simulink model "ExperimentalCarrier"  (R2015b)
settings: Solver=ode45  StartTime=0.0  StopTime=60  FixedStep=0.001  RelTol=1e-4
model workspace (MAT data in the model file):
  CX = [-0.0973267994662 -0.079334770792 -0.063312708602 -0.0492783817904 -0.0372483838751 -0.0272381795582 -0.0192622767468 -0.0133348794834 -0.00947247058383 -0.00770460619817 -0.00779177365154 -0.010332184952 ... (651 elements, 31x21)]
  CX_P = [0.00223913348595 0.00226279846593 0.00215584206323 0.00191826427785 0.0015500651098 0.00105124455907 0.000421802625665 -0.000338260690416 -0.00122894538917 -0.00225025147061 -0.00340217893471 -0.0046847277815 ... (651 elements, 31x21)]
  CX_Q = [0.566750126524 0.513799273419 0.46074149597 0.407560115115 0.354235092058 0.300738098816 0.247021798665 0.193002362465 0.138579422321 0.0841448328254 0.0156800910173 -0.028587220216 ... (651 elements, 31x21)]
  CX_R = [0.00872473439328 0.00961108484928 0.0104908055113 0.0113660862689 0.0122394567236 0.0131139410899 0.0139934759578 0.0148843304351 0.0158005787982 0.0167844985256 0.0173214701743 0.0192824833308 ... (651 elements, 31x21)]
  CX_d_elevator = [0.029681120923 0.0264274948833 0.0231424780296 0.019826833889 0.0164811360769 0.0131055318554 0.00969907215747 0.00625794011772 0.00277062099267 -0.000820697586383 -0.00752061307428 -0.00815142995882 ... (651 elements, 31x21)]
  CX_d_rudder = [-0.00683814731464 -0.00579287968011 -0.00473313798197 -0.00365917618136 -0.00257115069818 -0.00146908461552 -0.000352779652782 0.000778396676178 0.0019254949791 0.00307845824922 0.00430777388103 0.00587395376473 ... (651 elements, 31x21)]
  CY = [0.0748502535538 0.0755645920384 0.0762601803819 0.076936530444 0.0775935707011 0.0782321665355 0.078855460083 0.0794722913019 0.0801051244106 0.0807983900173 0.0815089407636 0.0810999911453 ... (651 elements, 31x21)]
  CY_P = [0.314314541533 0.314908852342 0.315908686179 0.317314043043 0.319124922936 0.321341325856 0.323963251804 0.32699070078 0.330423672784 0.334262167815 0.338506185874 0.343155726961 ... (651 elements, 31x21)]
  CY_Q = [0.206845108985 0.212153285689 0.217549246201 0.223041221006 0.22863865097 0.234352353828 0.240194164072 0.246174375163 0.252295596359 0.258590970539 0.26593702078 0.276814416222 ... (651 elements, 31x21)]
  CY_R = [-0.299983586918 -0.303050767939 -0.30608450573 -0.309088417238 -0.312066630946 -0.315024477354 -0.317970440697 -0.320921537604 -0.323916102322 -0.327010675103 -0.329661903523 -0.331314720608 ... (651 elements, 31x21)]
  CY_d_elevator = [0.0241602483601 0.024862141616 0.0255735782381 0.0262950172254 0.0270270636195 0.0277705820366 0.0285269750226 0.0292988478742 0.0300914026037 0.030913435532 0.0317596917419 0.0324941126108 ... (651 elements, 31x21)]
  CY_d_rudder = [-0.129392052709 -0.131156233114 -0.132888496587 -0.13458992916 -0.13626179938 -0.137905650351 -0.139523580046 -0.141119005177 -0.142698155317 -0.144262742569 -0.145575423934 -0.146927528452 ... (651 elements, 31x21)]
  CZ = [-0.635288026255 -0.561513437672 -0.486937541039 -0.411613157493 -0.335593450001 -0.258932000134 -0.181683022099 -0.10390236702 -0.025657439009 0.0528154193638 0.128636653723 0.209168379022 ... (651 elements, 31x21)]
  CZ_P = [-0.0426180741921 -0.040371283283 -0.0379977363135 -0.0354974332835 -0.0328703741931 -0.0301165590423 -0.027235987831 -0.0242286605594 -0.0210945772272 -0.0178337378347 -0.0144461423817 -0.0109317908683 ... (651 elements, 31x21)]
  CZ_Q = [6.96025865077 6.98114129849 7.00206820292 7.02304903766 7.04409127039 7.06519952703 7.08637371713 7.10760603499 7.12891815552 7.15129935899 7.15392062661 7.18837906802 ... (651 elements, 31x21)]
  CZ_R = [-0.105405414656 -0.106545289739 -0.107737293614 -0.108987554898 -0.110302712806 -0.111690005069 -0.113157533015 -0.114714527104 -0.116362189514 -0.11786971515 -0.114666901886 -0.118318379275 ... (651 elements, 31x21)]
  CZ_d_elevator = [0.51008994796 0.512918903365 0.515635142398 0.518238988463 0.520730557555 0.523109824579 0.525376856974 0.527532585768 0.529582683355 0.53158310039 0.53222009415 0.532991323176 ... (651 elements, 31x21)]
  CZ_d_rudder = [-0.0994246348718 -0.101114338005 -0.102795749856 -0.104468657243 -0.106132886268 -0.107788391525 -0.109435540346 -0.111075916846 -0.112714334729 -0.114363388416 -0.115472857798 -0.116943666826 ... (651 elements, 31x21)]
  Cl = [-0.0385814765962 -0.0383389644596 -0.0380848835968 -0.0378195009591 -0.0375431159662 -0.0372560730473 -0.0369588021987 -0.0366519368415 -0.0363364206354 -0.0360097812088 -0.0355885143095 -0.0352015390645 ... (651 elements, 31x21)]
  Cl_P = [-0.410096776624 -0.411715869817 -0.413321511523 -0.414913701743 -0.416492440476 -0.418057727723 -0.419609563483 -0.421147947757 -0.422672880544 -0.424184361845 -0.425682391659 -0.427166969987 ... (651 elements, 31x21)]
  Cl_Q = [0.0121734873015 0.0115511634771 0.0109219874117 0.0102856172191 0.00964162351347 0.00898936687588 0.00832771640535 0.00765433243871 0.00696211625156 0.00619409954578 0.00511750960358 0.00438446572798 ... (651 elements, 31x21)]
  Cl_R = [0.0639194118456 0.0641980766094 0.0644722880685 0.0647423901469 0.0650087480028 0.0652717875848 0.0655321272397 0.0657909713502 0.0660509927516 0.066314134037 0.0664428977346 0.0665956593355 ... (651 elements, 31x21)]
  Cl_d_elevator = [-0.00083845092376 -0.000897333841468 -0.000957239499541 -0.00101816580014 -0.00108011314323 -0.00114310126406 -0.00120721661945 -0.00127274325287 -0.00134057483614 -0.00141463059496 -0.00150116458646 -0.00150417720092 ... (651 elements, 31x21)]
  Cl_d_rudder = [0.0120074370195 0.0121224981409 0.0122343776715 0.0123431699853 0.0124489831282 0.0125519544191 0.0126522973225 0.0127504304685 0.0128472820476 0.012944583953 0.0130167454048 0.0130728202844 ... (651 elements, 31x21)]
  Cm = [0.0973465601848 0.0882383997807 0.0791321401801 0.0700083578182 0.060846163509 0.0516235998805 0.0423185376691 0.03291173616 0.0234098703618 0.0141912971055 0.0115389891247 -0.00108731819606 ... (651 elements, 31x21)]
  Cm_P = [0.204940910369 0.202805913545 0.20033190145 0.197518874086 0.194366831451 0.190875773546 0.187045700371 0.182876611925 0.17836850821 0.173521389224 0.168335254967 0.162810105441 ... (651 elements, 31x21)]
  Cm_Q = [-8.8302811579 -8.84673802608 -8.86380445529 -8.8815160128 -8.89990381522 -8.91899396376 -8.93880586357 -8.95935222087 -8.98073821097 -9.00528706826 -8.98625605481 -9.03648930164 ... (651 elements, 31x21)]
  Cm_R = [0.231203964913 0.23319997533 0.235299090374 0.237514849258 0.239861907942 0.242356170567 0.245015146547 0.247857975971 0.250885037596 0.253592063858 0.24580144055 0.252971901877 ... (651 elements, 31x21)]
  Cm_d_elevator = [-1.16934045694 -1.17556162403 -1.1814926709 -1.18713462751 -1.19248809506 -1.19755345312 -1.20233156667 -1.2068260282 -1.21105317786 -1.21514844284 -1.21623242778 -1.21673947768 ... (651 elements, 31x21)]
  Cm_d_rudder = [0.221327907125 0.224938352672 0.228521302045 0.232076418337 0.235603478751 0.239102604189 0.24257498777 0.246024952347 0.249465016904 0.252925369172 0.255135515483 0.258069205799 ... (651 elements, 31x21)]
  Cn = [0.0239084920706 0.0233651881183 0.0228219583067 0.0222793256831 0.0217379864069 0.0211990203144 0.0206644263801 0.0201384574022 0.0196305829364 0.0191582088364 0.0187126782059 0.0177875778536 ... (651 elements, 31x21)]
  Cn_P = [0.00271348744888 0.000830692215513 -0.000879092281498 -0.00241586604216 -0.00377962906647 -0.00497038135443 -0.00598812290603 -0.00683285372129 -0.0075045738002 -0.00800328314275 -0.00832898174895 -0.0084816696188 ... (651 elements, 31x21)]
  Cn_Q = [0.0646895607463 0.0668587351559 0.0690696353792 0.0713263026419 0.0736328941188 0.0759930959236 0.078408543068 0.0808750323066 0.0833760949483 0.0858871158776 0.0879312223138 0.0933690960242 ... (651 elements, 31x21)]
  Cn_R = [-0.107505906228 -0.108368888514 -0.109223762874 -0.110071896296 -0.110914888897 -0.111754897972 -0.112595502998 -0.113443913399 -0.114315599189 -0.115230945783 -0.115971844659 -0.116177724127 ... (651 elements, 31x21)]
  Cn_d_elevator = [0.00836627067687 0.00863561072168 0.00890974810625 0.00918895143726 0.009473528048 0.00976381947702 0.0100601758992 0.0103628424776 0.0106713097064 0.0109780163579 0.011109463637 0.0115746093706 ... (651 elements, 31x21)]
  Cn_d_rudder = [-0.0546400598137 -0.0553510121202 -0.0560495856635 -0.0567362885882 -0.0574116958811 -0.0580764807608 -0.0587315154598 -0.0593781486964 -0.060018716409 -0.060653217797 -0.0611661774955 -0.061673059209 ... (651 elements, 31x21)]
  aircraft_geometry_name = 'ExperimentalCarrier'
  alpha = [-0.174532925199; -0.157079632679; -0.13962634016; -0.12217304764; -0.10471975512; -0.0872664625997; -0.0698131700798; -0.0523598775598; -0.0349065850399; -0.0174532925199; 0; 0.0174532925199; 0.0349065850399; 0.0523598775598; 0.0698131700798; 0.0872664625997; 0.10471975512; 0.12217304764; 0.13962634016; 0.157079632679; 0.174532925199; 0.191986217719; 0.209439510239; 0.226892802759; 0.244346095279; 0.261799387799; 0.279252680319; 0.296705972839; 0.314159265359; 0.331612557879; 0.349065850399]
  beta = [-0.174532925199; -0.157079632679; -0.13962634016; -0.12217304764; -0.10471975512; -0.0872664625997; -0.0698131700798; -0.0523598775598; -0.0349065850399; -0.0174532925199; 0; 0.0174532925199; 0.0349065850399; 0.0523598775598; 0.0698131700798; 0.0872664625997; 0.10471975512; 0.12217304764; 0.13962634016; 0.157079632679; 0.174532925199]
  centerOfGravity = -0.092
  mass = 1.56
  mean_chord = 0.25
  spanwidth = 1.5
undefined symbols (not defined in the file): Earth, WGS84
libraries: aerolibconvert2 x6, aerolibnav x3, aerolibasang x2, aerolibfltsims x2, aerolib6dof2 x1, aerolibadyn x1, aerolibtransform2 x1, aerolibanimutils x1, aerolibatmos2 x1, aerolibgravity2 x1
(part 1 of 2)
settings Model: Creator=jruesch  LastModifiedBy=jruesch
settings DataIOCC: SaveFormat=Array
settings OptimizationCC: BlockReduction=off
settings HardwareCC: ProdBitPerPointer=32  ProdLargestAtomicFloat=None  ProdIntDivRoundTo=Undefined  ProdEndianess=Unspecified  ProdWordSize=32  ProdHWDeviceType=32-bit Generic
settings GRTTargetCC: GeneratePreprocessorConditionals=Disable all
settings ConfigComp: CovModelRefEnable=Off

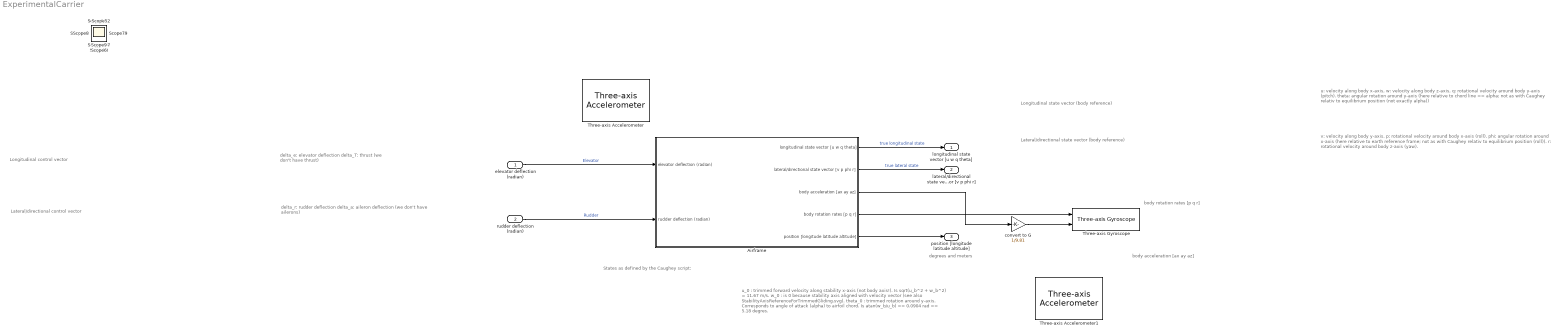
== system ExperimentalCarrier ==
  note: body acceleration [ax ay az]
  note: body rotation rates [p q r]
  note: degrees and meters
  note: States as defined by the Caughey script:
  note: u_0 : trimmed forward velocity along stability x-axis (not body axis!).
      | Is sqrt(u_b^2 + w_b^2) = 11.67 m/s.
      | w_0 : is 0 because stability axis aligned with velocity vector
      | (see also StabilityAxisReferenceForTrimmedGliding.svg).
      | theta_0 : trimmed rotation around y-axis. Corresponds
      | to angle of attack (alpha) to airfoil chord.
      | Is atan(w_b/u_b) == 0.0904 rad == 5.18 degres.
  note: delta_r: rudder deflection
      | delta_a: aileron deflection (we don't have ailerons)
  note: Lateral/directional control vector
  note: delta_e: elevator deflection
      | delta_T: thrust (we don't have thrust)
  note: Longitudinal control vector
  note: v: velocity along body y-axis.
      | p: rotational velocity around body x-axis (roll).
      | phi: angular rotation around x-axis (here relative to earth reference frame; not as with Caughey relativ to equilibrium position (roll)).
      | r: rotational velocity around body z-axis (yaw).
  note: u: velocity along body x-axis,
      | w: velocity along body z-axis,
      | q: rotational velocity around body y-axis (pitch).
      | theta: angular rotation around y-axis (here relative to chord line == alpha; not as with Caughey relativ to equilibrium position (not exactly alpha))
  note: Lateral/directional state vector (body reference)
  note: Longitudinal state vector (body reference)
  elevator deflection (radian) : Inport
  rudder deflection (radian) : Inport  Port=2
  Airframe : Subsystem
      mask Display: image(imread('../../figures/Airframe.png'))
  Three-axis Accelerometer : aerolibnav/Three-axis Accelerometer  units=Metric (MKS)  acc=[0 0 0]  gtype=on  dtype_a=on  w_a=190  z_a=0.707  a_sf_cc=[1 0 0; 0 1 0; 0 0 1]  a_bias=[0 0 0]  a_Ts=0  a_rand=on  a_seeds=[23093 23094 23095]  a_pow=[0.001 0.001 0.001]  a_sat="[-inf  -inf  -inf  inf inf inf]"
  Three-axis Accelerometer1 : aerolibnav/Three-axis Accelerometer  units=Metric (MKS)  acc=[0 0 0]  gtype=on  dtype_a=on  w_a=190  z_a=0.707  a_sf_cc=[1 0 0; 0 1 0; 0 0 1]  a_bias=[0 0 0]  a_Ts=0  a_rand=on  a_seeds=[23093 23094 23095]  a_pow=[0.001 0.001 0.001]  a_sat="[-inf  -inf  -inf  inf inf inf]"
  Three-axis Gyroscope : aerolibnav/Three-axis Gyroscope  dtype_g=on  w_g=190  z_g=0.707  g_sf_cc=[1 0 0; 0 1 0; 0 0 1]  g_bias=[0 0 0]  g_sen=[0 0 0]  g_Ts=0  g_rand=on  g_seeds=[23093 23094 23095]  g_pow=[0.0001 0.0001 0.0001]  g_sat="[-inf  -inf  -inf  inf inf inf]"
  convert to G : Gain  Gain=1/9.81
  longitudinal state vector [u w q theta] : Outport
  lateral/directional state vector [v p phi r] : Outport  Port=2
  position [longitude latitude altitude] : Outport  Port=3
  Scope{,1..40} (41 alike) : Scope
  wires:
  elevator deflection (radian)/1 -> Airframe/1(elevator deflection (radian))  "Elevator"
  rudder deflection (radian)/1 -> Airframe/2(rudder deflection (radian))  "Rudder"
  Airframe/1(longitudinal state vector [u w q theta]) -> longitudinal state vector [u w q theta]/1  "true longitudinal state"
  Airframe/2(lateral/directional state vector [v p phi r]) -> lateral/directional state vector [v p phi r]/1  "true lateral state"
  Airframe/3(body acceleration [ax ay az]) -> convert to G/1
  Airframe/4(body rotation rates [p q r]) -> Three-axis Gyroscope/1
  Airframe/5(position [longitude latitude altitude]) -> position [longitude latitude altitude]/1
  convert to G/1 -> Three-axis Gyroscope/2
